simulink model "TRAS_2dof_model"  (Simulink 7.7)
settings: Solver=ode14x  StartTime=0.0  StopTime=120  FixedStep=0.01  RelTol=1e-3
PreLoadFcn:
  | load tras_char
values from neighbouring files (symbols this model uses):
  Ad = Kd.A    [dms_tras.m]
  Bd = Kd.B    [dms_tras.m]
  Cd = Kd.C    [dms_tras.m]
  Dd = Kd.D    [dms_tras.m]
undefined symbols (not defined in the file or in its folder): control_a, control_p, force_a, force_p, rpm_a, rpm_p
settings Model: Creator=Petko Petkov  LastModifiedBy=Petko Petkov
settings DataIOCC: SignalLoggingName=sigsOut
settings OptimizationCC: InitFltsAndDblsToZero=on
settings DebuggingCC: SaveWithParameterizedLinksMsg=none  SignalResolutionControl=TryResolveAllWithWarning  SolverPrmCheckMsg=none  MultiTaskDSMMsg=warning  MultiTaskCondExecSysMsg=none  StrictBusMsg=None
settings HardwareCC: TargetEndianess=LittleEndian  TargetHWDeviceType=MATLAB Host  ProdEqTarget=off
settings RTWCC: IncludeERTFirstTime=on
settings GRTTargetCC: TargetFcnLib=ansi_tfl_tmw.mat

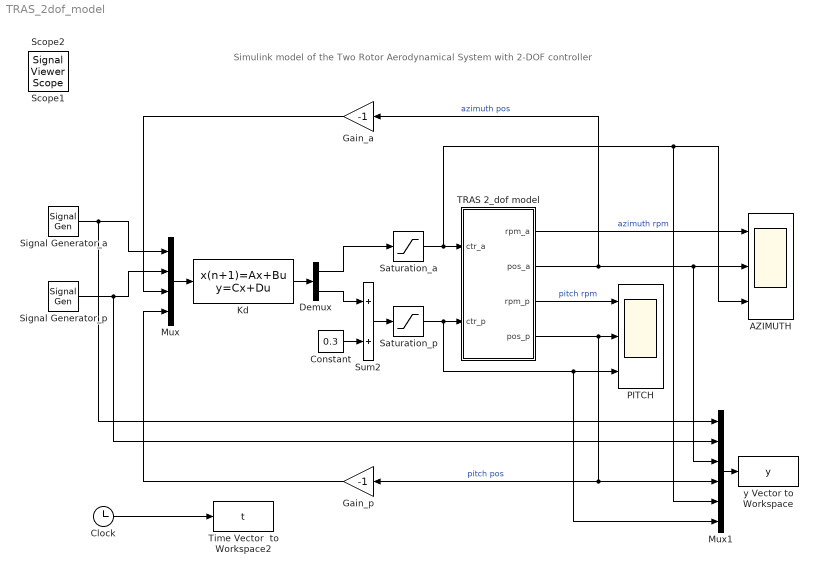
== system TRAS_2dof_model ==
  note: Simulink model of the Two Rotor Aerodynamical System with 2-DOF controller
  AZIMUTH : Scope  NumInputPorts=3
      settings: TimeRange=120  YMin=-3000~-0.4~-0.4  YMax=2000~0.4~0.3  MaxDataPoints=100000
  Clock : Clock
  Constant : Constant  Value=0.3
  Demux : Demux  Outputs=2
  Gain_a : Gain  Gain=-1
  Gain_p : Gain  Gain=-1
  Kd : DiscreteStateSpace  A=Ad  B=Bd  C=Cd  D=Dd  SampleTime=0.01
  Mux : Mux
  Mux1 : Mux  Inputs=6
  PITCH : Scope  NumInputPorts=3
      settings: TimeRange=120  YMin=0~-1~0.25  YMax=3000~0.5~0.45  MaxDataPoints=100000
  Saturation_a : Saturate  UpperLimit=0.8  LowerLimit=-0.8
  Saturation_p : Saturate  UpperLimit=1.0
  Signal Generator_a : SignalGenerator  WaveForm=square  Amplitude=0.4  Frequency=0.02
  Signal Generator_p : SignalGenerator  WaveForm=square  Amplitude=0.1  Frequency=1/60
  Sum2 : Sum  SaturateOnIntegerOverflow=on
  "TRAS 2_dof model " : Subsystem
  Time Vector  to Workspace2 : ToWorkspace  VariableName=t  SampleTime=-1  SaveFormat=Array
  y Vector to Workspace : ToWorkspace  VariableName=y  SampleTime=-1  SaveFormat=Array
  Scope1 : SignalViewerScope  IOType=viewer  RefreshTime=0.035000
  Scope2 : SignalViewerScope  IOType=viewer  RefreshTime=0.035000
  wires:
  "TRAS 2_dof model "/1(rpm_a) -> AZIMUTH/1  "azimuth rpm"
  "TRAS 2_dof model "/2(pos_a) -> Gain_a/1, AZIMUTH/2, Mux1/3  "azimuth pos"
  "TRAS 2_dof model "/3(rpm_p) -> PITCH/1  "pitch rpm"
  "TRAS 2_dof model "/4(pos_p) -> PITCH/2, Gain_p/1, Mux1/4  "pitch pos"
  Kd/1 -> Demux/1
  Mux/1 -> Kd/1
  Demux/1 -> Saturation_a/1
  Saturation_a/1 -> "TRAS 2_dof model "/1(ctr_a), AZIMUTH/3, Mux1/5
  Saturation_p/1 -> "TRAS 2_dof model "/2(ctr_p), PITCH/3, Mux1/6
  Sum2/1 -> Saturation_p/1
  Constant/1 -> Sum2/2
  Gain_a/1 -> Mux/3
  Gain_p/1 -> Mux/4
  Signal Generator_a/1 -> Mux/1, Mux1/1
  Signal Generator_p/1 -> Mux/2, Mux1/2
  Demux/2 -> Sum2/1
  Clock/1 -> Time Vector  to Workspace2/1
  Mux1/1 -> y Vector to Workspace/1

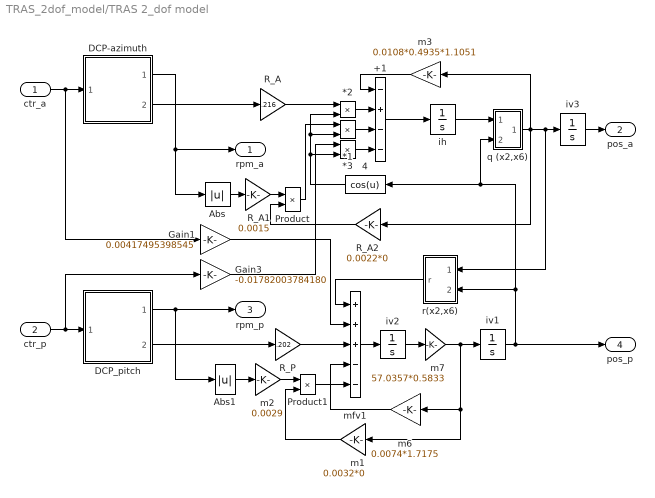
== system TRAS_2dof_model/TRAS 2_dof model  ==
  ctr_a : Inport
  ctr_p : Inport  Port=2
  *1 : Product  SaturateOnIntegerOverflow=on  InputSameDT=on  OutDataTypeStr=Inherit: Same as first input
  *2 : Product  SaturateOnIntegerOverflow=on  InputSameDT=on  OutDataTypeStr=Inherit: Same as first input
  *3 : Product  SaturateOnIntegerOverflow=on  InputSameDT=on  OutDataTypeStr=Inherit: Same as first input
  +1 : Sum  Inputs=-+--  SaturateOnIntegerOverflow=on  InputSameDT=on  OutDataTypeStr=Inherit: Same as first input
  4 : Fcn  Expr=cos(u)
  Abs : Abs  SaturateOnIntegerOverflow=on
  Abs1 : Abs  SaturateOnIntegerOverflow=on
  DCP-azimuth : Subsystem
  DCP_pitch : Subsystem
  Gain1 : Gain  Gain=0.00417495398545  SaturateOnIntegerOverflow=on  OutDataTypeStr=Inherit: Same as input  ParamDataTypeStr=Inherit: Same as input
  Gain3 : Gain  Gain=-0.01782003784180  SaturateOnIntegerOverflow=on  OutDataTypeStr=Inherit: Same as input  ParamDataTypeStr=Inherit: Same as input
  Product : Product  SaturateOnIntegerOverflow=on  InputSameDT=on  OutDataTypeStr=Inherit: Same as first input
  Product1 : Product  SaturateOnIntegerOverflow=on  OutDataTypeStr=Inherit: Same as first input
  R_A : Gain  Gain=.216  OutDataTypeStr=Inherit: Same as input  ParamDataTypeStr=Inherit: Same as input
  R_A1 : Gain  Gain=0.0015  OutDataTypeStr=Inherit: Same as input  ParamDataTypeStr=Inherit: Same as input
  R_A2 : Gain  Gain=0.0022*0  OutDataTypeStr=Inherit: Same as input  ParamDataTypeStr=Inherit: Same as input
  R_P : Gain  Gain=.202  OutDataTypeStr=Inherit: Same as input  ParamDataTypeStr=Inherit: Same as input
  ih : Integrator  UpperSaturationLimit=10  LowerSaturationLimit=-10
  iv1 : Integrator  InitialCondition=-0.2899  LimitOutput=on  UpperSaturationLimit=pi/2  LowerSaturationLimit=-pi/2
  iv2 : Integrator  UpperSaturationLimit=pi  LowerSaturationLimit=-pi
  iv3 : Integrator  InitialCondition=0.1795  LimitOutput=on  UpperSaturationLimit=6  LowerSaturationLimit=-6
  m1 : Gain  Gain=0.0032*0  SaturateOnIntegerOverflow=on  OutDataTypeStr=Inherit: Same as input  ParamDataTypeStr=Inherit: Same as input
  m2 : Gain  Gain=0.0029  SaturateOnIntegerOverflow=on  OutDataTypeStr=Inherit: Same as input  ParamDataTypeStr=Inherit: Same as input
  m3 : Gain  Gain=0.0108*0.4935*1.1051  OutDataTypeStr=Inherit: Same as input  ParamDataTypeStr=Inherit: Same as input
  m6 : Gain  Gain=0.0074*1.7175  OutDataTypeStr=Inherit: Same as input  ParamDataTypeStr=Inherit: Same as input
  m7 : Gain  Gain=57.0357*0.5833  SaturateOnIntegerOverflow=on  OutDataTypeStr=Inherit: Same as input  ParamDataTypeStr=Inherit: Same as input
  mfv1 : Sum  Inputs=+++--  SaturateOnIntegerOverflow=on  InputSameDT=on  OutDataTypeStr=Inherit: Same as first input
  q (x2,x6) : Subsystem
  r(x2,x6) : Subsystem
  rpm_a : Outport
  pos_a : Outport  Port=2
  rpm_p : Outport  Port=3
  pos_p : Outport  Port=4
  wires:
  DCP-azimuth/2(FORCE_A) -> R_A/1
  *1/1 -> +1/3
  m3/1 -> +1/1
  *2/1 -> +1/2
  ih/1 -> q (x2,x6)/1(x2)
  q (x2,x6)/1(q) -> iv3/1, r(x2,x6)/1(y2), m3/1, R_A2/1
  R_A/1 -> *2/1
  Abs/1 -> R_A1/1
  R_A1/1 -> Product/1
  R_A2/1 -> Product/2
  DCP_pitch/2(FORCE_P) -> R_P/1
  m6/1 -> mfv1/4
  iv2/1 -> m7/1
  mfv1/1 -> iv2/1
  m7/1 -> iv1/1, m6/1, m1/1
  DCP_pitch/1(RPM_P) -> Abs1/1, rpm_p/1
  Abs1/1 -> m2/1
  Product1/1 -> mfv1/5
  r(x2,x6)/1(r) -> mfv1/1
  R_P/1 -> mfv1/3
  iv1/1 -> pos_p/1, r(x2,x6)/2(x6), 4/1, q (x2,x6)/2(x6)
  m1/1 -> Product1/2
  m2/1 -> Product1/1
  *3/1 -> +1/4
  Product/1 -> *1/1
  4/1 -> *2/2, *1/2, *3/2
  Gain1/1 -> mfv1/2
  Gain3/1 -> *3/1
  ctr_a/1 -> DCP-azimuth/1(CTR_A), Gain1/1
  ctr_p/1 -> DCP_pitch/1(CTR_P), Gain3/1
  iv3/1 -> pos_a/1
  +1/1 -> ih/1
  DCP-azimuth/1(RPM_A) -> rpm_a/1, Abs/1

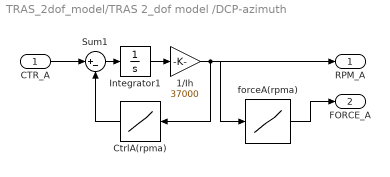
== system TRAS_2dof_model/TRAS 2_dof model /DCP-azimuth ==
  CTR_A : Inport
  1/Ih : Gain  Gain=37000  SaturateOnIntegerOverflow=on  OutDataTypeStr=Inherit: Same as input  ParamDataTypeStr=Inherit: Same as input
  CtrlA(rpma) : Lookup  InputValues=rpm_a  Table=control_a  SaturateOnIntegerOverflow=on
  Integrator1 : Integrator
  Sum1 : Sum  Inputs=|+-  SaturateOnIntegerOverflow=on  InputSameDT=on  OutDataTypeStr=Inherit: Same as first input
  forceA(rpma) : Lookup  InputValues=rpm_a  Table=force_a  SaturateOnIntegerOverflow=on
  RPM_A : Outport
  FORCE_A : Outport  Port=2
  wires:
  Sum1/1 -> Integrator1/1
  CtrlA(rpma)/1 -> Sum1/2
  Integrator1/1 -> 1/Ih/1
  1/Ih/1 -> CtrlA(rpma)/1, forceA(rpma)/1, RPM_A/1
  CTR_A/1 -> Sum1/1
  forceA(rpma)/1 -> FORCE_A/1

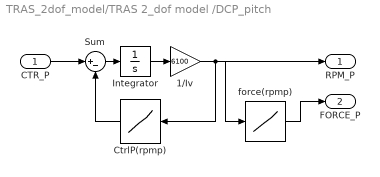
== system TRAS_2dof_model/TRAS 2_dof model /DCP_pitch ==
  CTR_P : Inport
  1/Iv : Gain  Gain=6100  OutDataTypeStr=Inherit: Same as input  ParamDataTypeStr=Inherit: Same as input
  CtrlP(rpmp) : Lookup  InputValues=rpm_p  Table=control_p  SaturateOnIntegerOverflow=on
  Integrator : Integrator
  Sum : Sum  Inputs=|+-  SaturateOnIntegerOverflow=on  InputSameDT=on  OutDataTypeStr=Inherit: Same as first input
  force(rpmp) : Lookup  InputValues=rpm_p  Table=force_p  SaturateOnIntegerOverflow=on
  RPM_P : Outport
  FORCE_P : Outport  Port=2
  wires:
  Sum/1 -> Integrator/1
  Integrator/1 -> 1/Iv/1
  CtrlP(rpmp)/1 -> Sum/2
  1/Iv/1 -> CtrlP(rpmp)/1, force(rpmp)/1, RPM_P/1
  CTR_P/1 -> Sum/1
  force(rpmp)/1 -> FORCE_P/1

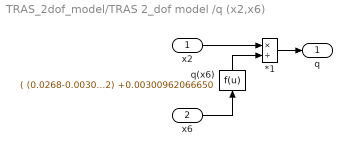
== system TRAS_2dof_model/TRAS 2_dof model /q (x2,x6) ==
  x2 : Inport
  x6 : Inport  Port=2
  " q(x6)" : Fcn  Expr=( (0.0268-0.00300962066650)*cos(u)^2) +0.00300962066650
  *1 : Product  Inputs=*/  SaturateOnIntegerOverflow=on  InputSameDT=on  OutDataTypeStr=Inherit: Same as first input
  q : Outport
  wires:
  *1/1 -> q/1
  x2/1 -> *1/1
  x6/1 -> " q(x6)"/1
  " q(x6)"/1 -> *1/2

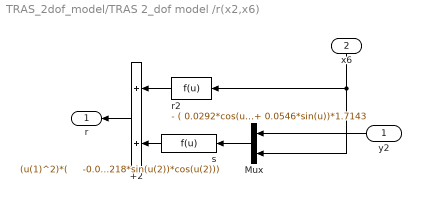
== system TRAS_2dof_model/TRAS 2_dof model /r(x2,x6) ==
  y2 : Inport
  x6 : Inport  Port=2
  +2 : Sum  SaturateOnIntegerOverflow=on  InputSameDT=on  OutDataTypeStr=Inherit: Same as first input
  Mux : Mux  Inputs=2
  r2 : Fcn  Expr=- ( 0.0292*cos(u)+ 0.0546*sin(u))*1.7143
  s : Fcn  Expr="(u(1)^2)*(     -0.07389953104162*  0.28753198180218*sin(u(2))*cos(u(2)))"
  r : Outport
  wires:
  Mux/1 -> s/1
  r2/1 -> +2/1
  s/1 -> +2/2
  x6/1 -> Mux/2, r2/1
  +2/1 -> r/1
  y2/1 -> Mux/1
